simulink model "Practica_control_ej_1_2_3"  (R2024b)
settings: Solver=VariableStepAuto  StartTime=0.0  StopTime=10  RelTol=1e-3
model workspace (MAT data in the model file):
  B2 = 2500
  k1 = 50000
  k2 = 1000
  m1 = 20
  m2 = 1300
settings Model: Creator=Carlos  LastModifiedBy=carlos

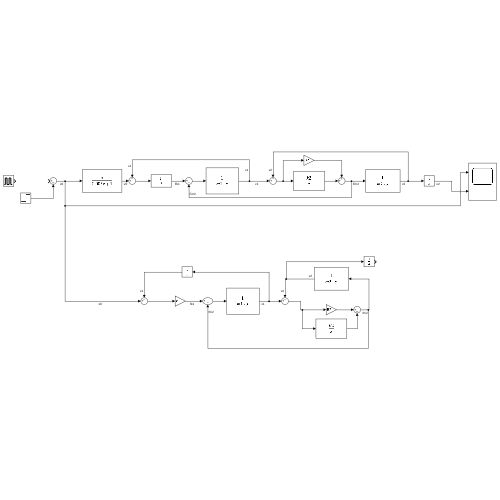
[thumbnail: Simulink's stored preview of the top-level diagram]
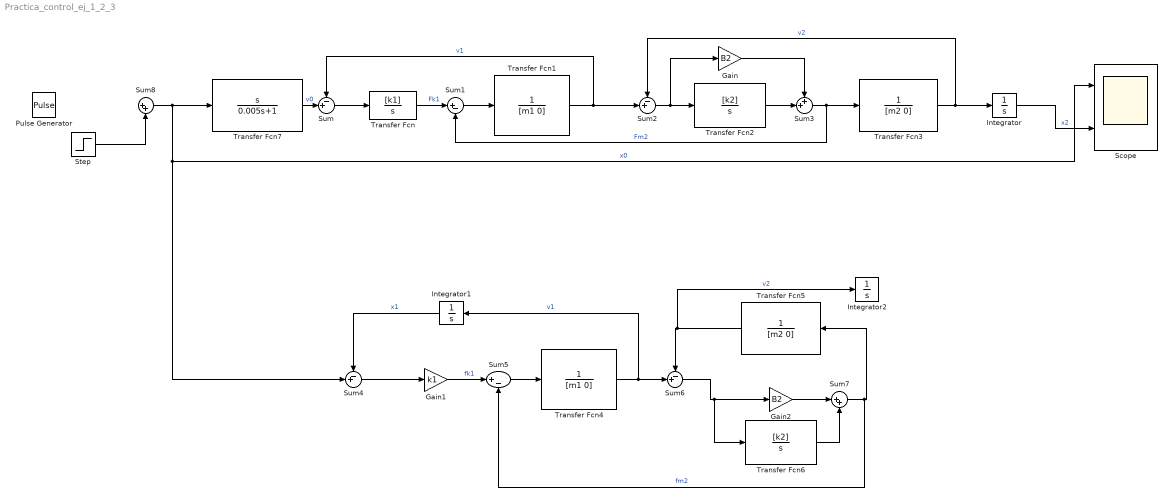
== system Practica_control_ej_1_2_3 ==
  Gain : Gain  Gain=B2
  Gain1 : Gain  Gain=k1
  Gain2 : Gain  Gain=B2
  Integrator : Integrator
  Integrator1 : Integrator
  Integrator2 : Integrator
  Pulse Generator : DiscretePulseGenerator  PulseType=Time based  Amplitude=0.1  Period=10  PulseWidth=10
  Scope : Scope  NumInputPorts=2
  Step : Step  After=0.1  SampleTime=0
  Sum{,2,4,6} (4 alike) : Sum  Inputs=-+|
  Sum1 : Sum  Inputs=|+-
  Sum3 : Sum  Inputs=++|
  Sum5 : Sum  Inputs=|+-
  Sum7 : Sum  Inputs=|++
  Sum8 : Sum  Inputs=|++
  Transfer Fcn : TransferFcn  Numerator=[k1]  Denominator=[1 0]
  Transfer Fcn1 : TransferFcn  Denominator=[m1 0]
  Transfer Fcn2 : TransferFcn  Numerator=[k2]  Denominator=[1 0]
  Transfer Fcn3 : TransferFcn  Denominator=[m2 0]
  Transfer Fcn4 : TransferFcn  Denominator=[m1 0]
  Transfer Fcn5 : TransferFcn  Denominator=[m2 0]
  Transfer Fcn6 : TransferFcn  Numerator=[k2]  Denominator=[1 0]
  Transfer Fcn7 : TransferFcn  Numerator=[1 0]  Denominator=[0.005 1]
  wires:
  Transfer Fcn1/1 -> Sum2/2, Sum/1  "v1"
  Sum/1 -> Transfer Fcn/1
  Transfer Fcn/1 -> Sum1/1  "Fk1"
  Sum3/1 -> Sum1/2, Transfer Fcn3/1  "Fm2"
  Sum1/1 -> Transfer Fcn1/1
  Transfer Fcn3/1 -> Sum2/1, Integrator/1  "v2"
  Sum2/1 -> Gain/1, Transfer Fcn2/1
  Transfer Fcn2/1 -> Sum3/2
  Gain/1 -> Sum3/1
  Gain1/1 -> Sum5/1  "fk1"
  Sum4/1 -> Gain1/1
  Sum5/1 -> Transfer Fcn4/1
  Transfer Fcn4/1 -> Integrator1/1, Sum6/2  "v1"
  Transfer Fcn5/1 -> Integrator2/1, Sum6/1  "v2"
  Sum6/1 -> Transfer Fcn6/1, Gain2/1
  Gain2/1 -> Sum7/1
  Transfer Fcn6/1 -> Sum7/2
  Sum7/1 -> Sum5/2, Transfer Fcn5/1  "fm2"
  Sum8/1 -> Scope/1, Sum4/2, Transfer Fcn7/1  "x0"
  Integrator1/1 -> Sum4/1  "x1"
  Integrator/1 -> Scope/2  "x2"
  Step/1 -> Sum8/2
  Transfer Fcn7/1 -> Sum/2  "v0"
